simulink model "FIR_DirectForm"  (R2020b)
settings: Solver=VariableStepAuto  StartTime=0.0  StopTime=10.0  RelTol=1e-3
settings Model: Creator=Admin  LastModifiedBy=Admin

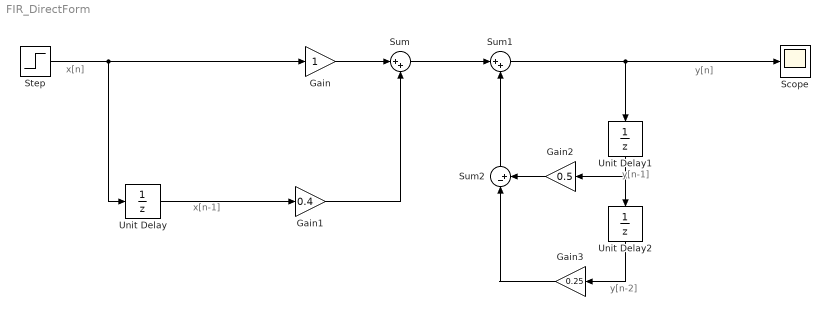
== system FIR_DirectForm ==
  note: y[n-1]
  note: y[n-2]
  note: x[n-1]
  note: x[n]
  note: y[n]
  Gain : Gain
  Gain1 : Gain  Gain=0.4
  Gain2 : Gain  Gain=0.5
  Gain3 : Gain  Gain=0.25
  Scope : Scope
  Step : Step  SampleTime=0
  Sum : Sum  Inputs=|++
  Sum1 : Sum  Inputs=|++
  Sum2 : Sum  Inputs=|-+
  Unit Delay : UnitDelay  SampleTime=-1  HasFrameUpgradeWarning=on
  Unit Delay1 : UnitDelay  SampleTime=-1  HasFrameUpgradeWarning=on
  Unit Delay2 : UnitDelay  SampleTime=-1  HasFrameUpgradeWarning=on
  wires:
  Unit Delay2/1 -> Gain3/1
  Sum1/1 -> Scope/1, Unit Delay1/1
  Sum2/1 -> Sum1/2
  Step/1 -> Unit Delay/1, Gain/1
  Gain1/1 -> Sum/2
  Gain3/1 -> Sum2/1
  Gain2/1 -> Sum2/2
  Sum/1 -> Sum1/1
  Unit Delay1/1 -> Gain2/1, Unit Delay2/1
  Unit Delay/1 -> Gain1/1
  Gain/1 -> Sum/1
